simulink model "Requriment_4"  (R2021a)
settings: Solver=FixedStepDiscrete  StartTime=0.0  StopTime=50  FixedStep=1  RelTol=1e-3
libraries: simulink x5
settings Model: Creator=Admin  LastModifiedBy=Rahul
settings SolverCC: AlgebraicLoopSolver=TrustRegion
settings OptimizationCC: DefaultParameterBehavior=Inlined  UseDivisionForNetSlopeComputation=on  EnhancedBackFolding=on  PassReuseOutputArgsAs=Individual arguments  OptimizeBlockOrder=speed  DifferentSizesBufferReuse=on  OptimizationCustomize=off  EfficientTunableParamExpr=on
settings DebuggingCC: SignalInfNanChecking=error  ParameterTunabilityLossMsg=error  UniqueDataStoreMsg=error  AssertControl=DisableAll  StrictBusMsg=ErrorOnBusTreatedAsVector  SFUndirectedBroadcastEventsDiag=error  SFMachineParentedDataDiag=warning
settings SFSimCC: CompileTimeRecursionLimit=0  EnableRuntimeRecursion=off  MATLABDynamicMemAlloc=off  CustomCodeUndefinedFunction=UseInterfaceOnly
settings RTWCC: SystemTargetFile=ert.tlc  TemplateMakefile=ert_default_tmf  GenerateReport=on  IncludeHyperlinkInReport=on  LaunchReport=on  GenerateTraceInfo=on  GenerateTraceReport=on  GenerateTraceReportSl=on  GenerateTraceReportSf=on  GenerateTraceReportEml=on
settings CodeAppCC: ForceParamTrailComments=on  IgnoreCustomStorageClasses=off  OperatorAnnotations=on  SimulinkDataObjDesc=on  SFDataObjDesc=on  MATLABFcnDesc=on  InsertBlockDesc=on
settings ERTTargetCC: TargetLangStandard=C99 (ISO)  UtilityFuncGeneration=Shared location  GenerateSampleERTMain=on  SupportNonFinite=off  ParenthesesLevel=Maximum  CastingMode=Standards  GenerateSharedConstants=off  InlinedParameterPlacement=NonHierarchical  ERTCustomFileTemplate=example_file_process.tlc  EnableSignedLeftShifts=off  EnableSignedRightShifts=off
settings ConfigComp: CovMetricSettings=dcmwe  PSAutoStubLUT=on

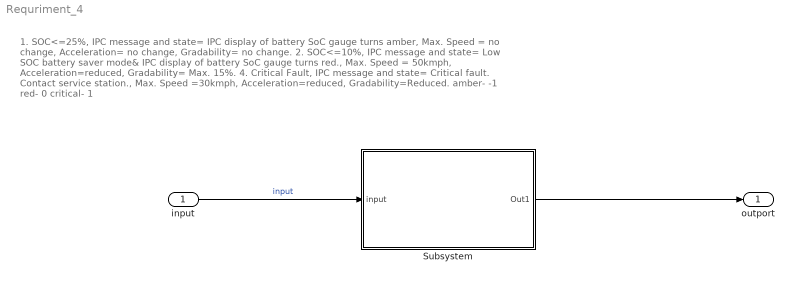
== system Requriment_4 ==
  note: 1. SOC<=25%, IPC message and state= IPC display of battery SoC gauge turns amber, Max. Speed = no change, Acceleration= no change, Gradability= no change.
      | 2. SOC<=10%, IPC message and state= Low SOC battery saver mode& IPC display of battery SoC gauge turns red., Max. Speed = 50kmph, Acceleration=reduced, Gradability= Max. 15%.
      | 4. Critical Fault, IPC message and state= Critical fault. Contact service station., Max. Speed =30kmph, Acceleration=reduced, Gradability=Reduced.
      | amber- -1 red- 0 critical- 1
  input : Inport
  Subsystem : Subsystem
  outport : Outport  VectorParamsAs1DForOutWhenUnconnected=off
  wires:
  input/1 -> Subsystem/1(input)  "input"
  Subsystem/1(Out1) -> outport/1

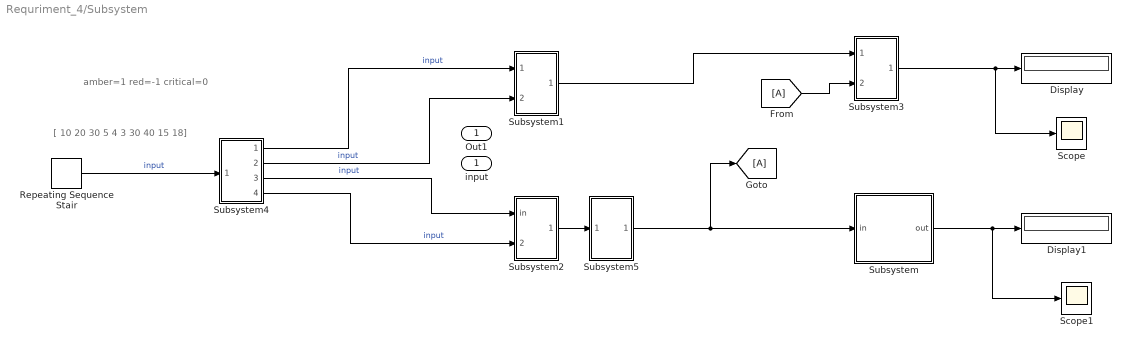
== system Requriment_4/Subsystem ==
  note: amber=1
      | red=-1
      | critical=0
  note: [ 10 20 30 5 4 3 30 40 15 18]
  input : Inport
  Display : Display
  Display1 : Display
  Repeating Sequence Stair : simulink/Sources/Repeating Sequence Stair  OutValues=[9 10 4 20 30 3 40 50 12 19 25 4]  tsamp=-1  OutMin=[]  OutMax=[]  OutDataTypeStr=double  OutputDataTypeScalingMode=double  OutDataType=fixdt(0,8)  ConRadixGroup=Best Precision: Vector-wise  OutScaling=2^-12
  Scope : Scope
  Scope1 : Scope
  Subsystem : Subsystem
  Subsystem1 : Subsystem
  Subsystem2 : Subsystem
  Subsystem3 : Subsystem
  Subsystem4 : Subsystem
  Subsystem5 : Subsystem
  Out1 : Outport  VectorParamsAs1DForOutWhenUnconnected=off
  wires:
  Subsystem1/1(out1) -> Subsystem3/1(In1)
  Subsystem3/1(output) -> Scope/1, Display/1
  Subsystem4/1(out1) -> Subsystem1/1(in1)  "input"
  Subsystem4/2(out2) -> Subsystem1/2(in2)  "input"
  Subsystem4/3(out3) -> Subsystem2/1(in)  "input"
  Subsystem4/4(out4) -> Subsystem2/2(input)  "input"
  Subsystem2/1(out1) -> Subsystem5/1(In1)
  Subsystem/1(out) -> Scope1/1, Display1/1
  Repeating Sequence Stair/1 -> Subsystem4/1(input1)  "input"
  Subsystem5/1(out) -> [A], Subsystem/1(in)
  [A] -> Subsystem3/2(inport)

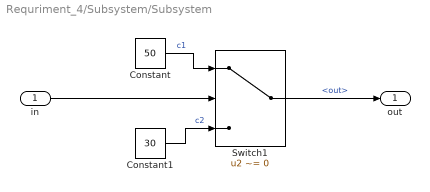
== system Requriment_4/Subsystem/Subsystem ==
  in : Inport
  Constant : Constant  Value=50
  Constant1 : Constant  Value=30
  Switch1 : Switch  Criteria=u2 ~= 0
  out : Outport  VectorParamsAs1DForOutWhenUnconnected=off
  wires:
  Constant/1 -> Switch1/1  "c1"
  Constant1/1 -> Switch1/3  "c2"
  in/1 -> Switch1/2
  Switch1/1 -> out/1  "<out>"

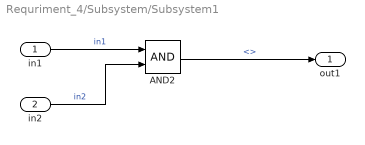
== system Requriment_4/Subsystem/Subsystem1 ==
  in1 : Inport
  in2 : Inport  Port=2
  AND2 : Logic  AllPortsSameDT=off  OutDataTypeStr=boolean
  out1 : Outport  VectorParamsAs1DForOutWhenUnconnected=off
  wires:
  AND2/1 -> out1/1  "<>"
  in1/1 -> AND2/1  "in1"
  in2/1 -> AND2/2  "in2"

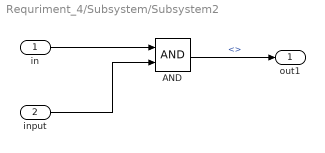
== system Requriment_4/Subsystem/Subsystem2 ==
  in : Inport
  input : Inport  Port=2
  AND : Logic  AllPortsSameDT=off  OutDataTypeStr=boolean
  out1 : Outport  VectorParamsAs1DForOutWhenUnconnected=off
  wires:
  input/1 -> AND/2
  in/1 -> AND/1
  AND/1 -> out1/1  "<>"

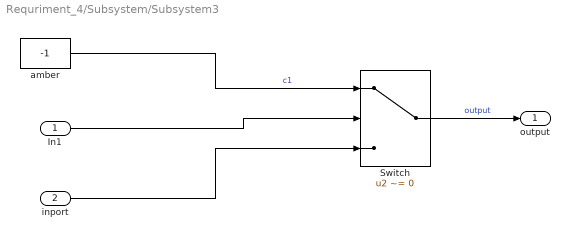
== system Requriment_4/Subsystem/Subsystem3 ==
  In1 : Inport
  inport : Inport  Port=2
  Switch : Switch  Criteria=u2 ~= 0
  amber : Constant  Value=-1
  output : Outport  VectorParamsAs1DForOutWhenUnconnected=off
  wires:
  amber/1 -> Switch/1  "c1"
  In1/1 -> Switch/2
  Switch/1 -> output/1  "output"
  inport/1 -> Switch/3

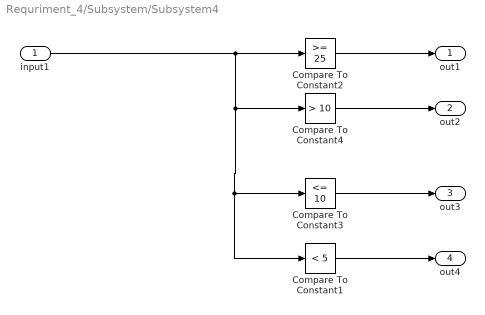
== system Requriment_4/Subsystem/Subsystem4 ==
  input1 : Inport
  Compare To Constant1 : simulink/Logic and Bit Operations/Compare To Constant  relop=<  const=5  OutDataTypeStr=boolean
  Compare To Constant2 : simulink/Logic and Bit Operations/Compare To Constant  relop=>=  const=25  OutDataTypeStr=boolean
  Compare To Constant3 : simulink/Logic and Bit Operations/Compare To Constant  relop=<=  const=10  OutDataTypeStr=boolean
  Compare To Constant4 : simulink/Logic and Bit Operations/Compare To Constant  relop=>  const=10  OutDataTypeStr=boolean
  out1 : Outport  VectorParamsAs1DForOutWhenUnconnected=off
  out2 : Outport  Port=2  VectorParamsAs1DForOutWhenUnconnected=off
  out3 : Outport  Port=3  VectorParamsAs1DForOutWhenUnconnected=off
  out4 : Outport  Port=4  VectorParamsAs1DForOutWhenUnconnected=off
  wires:
  Compare To Constant2/1 -> out1/1
  Compare To Constant1/1 -> out4/1
  input1/1 -> Compare To Constant1/1, Compare To Constant3/1, Compare To Constant4/1, Compare To Constant2/1
  Compare To Constant4/1 -> out2/1
  Compare To Constant3/1 -> out3/1

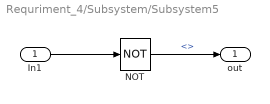
== system Requriment_4/Subsystem/Subsystem5 ==
  In1 : Inport
  NOT : Logic  Operator=NOT  IconShape=distinctive  AllPortsSameDT=off  OutDataTypeStr=boolean
  out : Outport  VectorParamsAs1DForOutWhenUnconnected=off
  wires:
  NOT/1 -> out/1  "<>"
  In1/1 -> NOT/1
